simulink model "testProject"  (R2023a)
settings: Solver=FixedStepDiscrete  StartTime=0.0  StopTime=inf  FixedStep=0.01  RelTol=1e-3
undefined symbols (not defined in the file): asdefe, erfwerf, gain, gStrOut, gStruInputs, MyInputsType, MyOutputType
libraries: bur_blks x4
settings Model: SimulationMode=external  Creator=stadelmanj  LastModifiedBy=stadelmanj
settings DataIOCC: SaveFormat=Array  SaveOutput=off  SignalLogging=off  DSMLogging=off  SaveTime=off  ReturnWorkspaceOutputs=off
settings OptimizationCC: DefaultParameterBehavior=Inlined  OptimizeBlockIOStorage=off  EnableMemcpy=off  ZeroExternalMemoryAtStartup=off  ZeroInternalMemoryAtStartup=off  InitFltsAndDblsToZero=on  LifeSpan=inf  OptimizeBlockOrder=speed  DifferentSizesBufferReuse=on  EfficientTunableParamExpr=on
settings DebuggingCC: UnderspecifiedInitializationDetection=Classic  MergeDetectMultiDrivingBlocksExec=none  SolverPrmCheckMsg=warning  InheritedTsInSrcMsg=none  FcnCallInpInsideContextMsg=warning  UnconnectedInputMsg=warning  UnconnectedOutputMsg=warning  UnconnectedLineMsg=warning  FrameProcessingCompatibilityMsg=none  ModelReferenceSymbolNameMessage=none  StateNameClashWarn=warning  SFUnexpectedBacktrackingDiag=warning  SFNoUnconditionalDefaultTransitionDiag=warning
settings HardwareCC: ProdBitPerPointer=32  ProdBitPerSizeT=32  ProdBitPerPtrDiffT=32  ProdLargestAtomicFloat=None  ProdWordSize=32  ProdHWDeviceType=Intel->x86/Pentium
settings ModelReferenceCC: UpdateModelReferenceTargets=IfOutOfDate  ModelReferencePassRootInputsByReference=off  PropagateSignalLabelsOutOfModel=off
settings SFSimCC: MATLABDynamicMemAlloc=off
settings RTWCC: Description=B&R Automation Studio Target (ERT based)  SystemTargetFile=bur_ert.tlc  GenerateMakefile=off  TemplateMakefile=bur.tmf  RTWVerbose=off
settings CodeAppCC: IgnoreTestpoints=on  CustomSymbolStrType=$N$R$M  InternalIdentifier=Classic
settings STFCustomTargetCC: MultiwordLength=256  ParMdlRefBuildCompliant=on  ConcurrentExecutionCompliant=off  ERTCustomFileBanners=on  SupportNonFinite=off  SupportNonInlinedSFcns=off  RemoveResetFunc=on  MATLABClassNameForMDSCustomization=Simulink.SoftwareTarget.ERTCustomization  GRTInterface=off  UseToolchainInfoCompliant=off  SystemTargetFile=bur_ert.tlc
settings ERTTargetCC: TargetLangStandard=C99 (ISO)  CompOptLevelCompliant=off  ConcurrentExecutionCompliant=off  CombineOutputUpdateFcns=off  SupportNonFinite=off  SupportContinuousTime=on  ModelStepFunctionPrototypeControlCompliant=off  CPPClassGenCompliant=off  UseToolchainInfoCompliant=off  ExtMode=on  ExtModeStaticAlloc=on  ExtModeMexArgs='127.0.0.1' 0 17724  InlinedParameterPlacement=NonHierarchical  MultiInstanceErrorCode=Warning  RootIOFormat=Part of model data structure  ERTSrcFileBannerTemplate=bur_code_c_template.cgt  ERTHdrFileBannerTemplate=bur_code_h_template.cgt  ERTDataSrcFileTemplate=bur_data_c_template.cgt  ERTDataHdrFileTemplate=bur_data_h_template.cgt  ERTCustomFileTemplate=bur_file_process.tlc  ConvertIfToSwitch=off  SuppressUnreachableDefaultCases=off

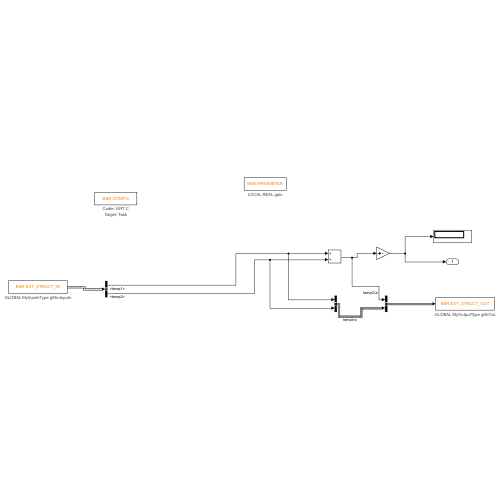
[thumbnail: Simulink's stored preview of the top-level diagram]
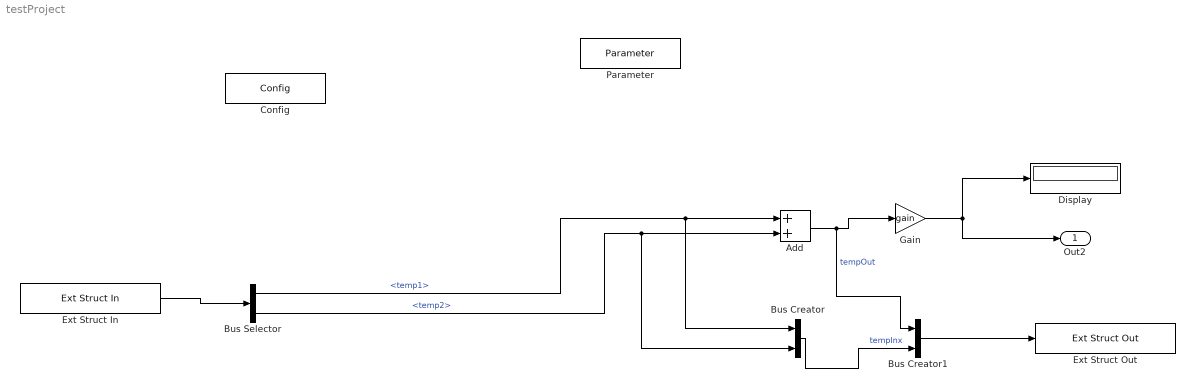
== system testProject ==
  Add : Sum
  Bus Creator : BusCreator  Inputs=2
  Bus Creator1 : BusCreator  Inputs=2
  Bus Selector : BusSelector  OutputSignals=temp1,temp2
  Config : bur_blks/Config  Tag=Coder: ERT C Target: Task  bur_configset_ert=C - Code Generation (Embedded Real Time Target based)  bur_configset_grt=C - Code Generation (Generic Real Time Target based)  bur_maskHandle=-1
      settings: AttributesFormatString=%<Tag>  SourceProductName=B&R Automation Studio Toolbox
  Display : Display
  Ext Struct In : bur_blks/Ext Struct In  Tag=GLOBAL MyInputsType gStruInputs  bur_var_name=gStruInputs  bur_var_description=erfwerf  bur_scope=GLOBAL  bur_var_memory=standard  bur_struct_name=MyInputsType  bur_AS_string=gStruInputs : MyInputsType; (*erfwerf*)  bur_AS_typ_list_string=MyInputsType
      settings: AttributesFormatString=%<Tag>  SourceProductName=B&R Automation Studio Toolbox
  Ext Struct Out : bur_blks/Ext Struct Out  Tag=GLOBAL MyOutputType gStrOut  bur_var_name=gStrOut  bur_var_description=asdefe  bur_scope=GLOBAL  bur_var_memory=standard  bur_struct_name=MyOutputType  bur_init_struct=[]  bur_AS_string=gStrOut : MyOutputType; (*asdefe*)  bur_AS_typ_list_string=MyOutputType Bus: MyInputsType
      settings: AttributesFormatString=%<Tag>  SourceProductName=B&R Automation Studio Toolbox
  Gain : Gain  Gain=gain
  Parameter : bur_blks/Parameter  Tag=LOCAL REAL gain  Priority=2147483646  bur_var_name=gain  bur_var_description=myGain  bur_scope=LOCAL  bur_data_type=REAL  bur_init_value=0.5  bur_init_value_bool=FALSE  bur_array_index=0  bur_old_var_name=Parameter1  bur_var_memory=standard  bur_array_index_string=1
      settings: AttributesFormatString=%<Tag>  SourceProductName=B&R Automation Studio Toolbox
  Out2 : Outport
  wires:
  Add/1 -> Bus Creator1/1, Gain/1  "tempOut"
  Gain/1 -> Out2/1, Display/1
  Bus Selector/1 -> Bus Creator/1, Add/1  "<temp1>"
  Bus Selector/2 -> Bus Creator/2, Add/2  "<temp2>"
  Ext Struct In/1 -> Bus Selector/1
  Bus Creator/1 -> Bus Creator1/2  "tempInx"
  Bus Creator1/1 -> Ext Struct Out/1
